simulink model "AE_315_W2_mass_spring_damper"  (R2022b)
settings: Solver=VariableStepAuto  StartTime=0.0  StopTime=10.0  RelTol=1e-3
settings Model: Creator=SoftLaptop  LastModifiedBy=SoftLaptop

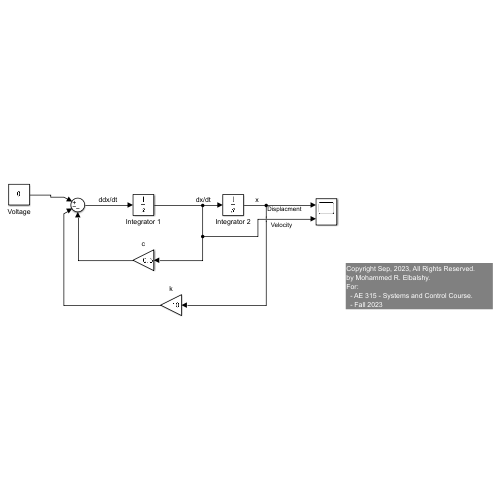
[thumbnail: Simulink's stored preview of the top-level diagram]
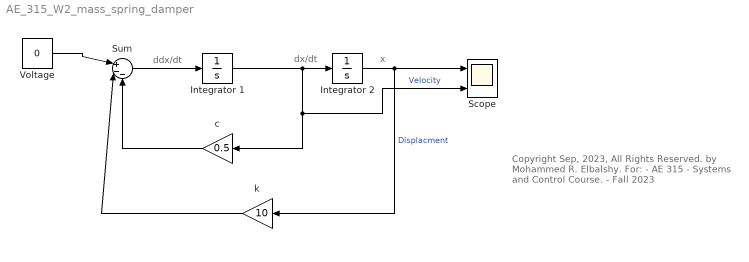
== system AE_315_W2_mass_spring_damper ==
  note: dx/dt
  note: x
  note: Copyright Sep, 2023, All Rights Reserved.
      | by Mohammed R. Elbalshy.
      | For:
      | - AE 315 - Systems and Control Course.
      | - Fall 2023
  note: ddx/dt
  Integrator 1 : Integrator  InitialCondition=1
  Integrator 2 : Integrator
  Scope : Scope  NumInputPorts=2
  Sum : Sum  Inputs=|+--
  Voltage : Constant  Value=0
  c : Gain  Gain=0.5
  k : Gain  Gain=10
  wires:
  c/1 -> Sum/3
  k/1 -> Sum/2
  Voltage/1 -> Sum/1
  Integrator 1/1 -> Scope/2, c/1, Integrator 2/1  "Velocity"
  Integrator 2/1 -> k/1, Scope/1  "Displacment"
  Sum/1 -> Integrator 1/1
